simulink model "wind_disturbance"  (R2016b)
settings: Solver=VariableStepAuto  StartTime=0.0  StopTime=10.0  RelTol=1e-3
values from neighbouring files (symbols this model uses):
  K = gain(x)    [radar_sweep.m]    (also in sweep.m; sweep_1.m; sweep_2.m; wind_sweep.m)
settings Model: Creator=ammar_laptop  LastModifiedBy=ammar_laptop

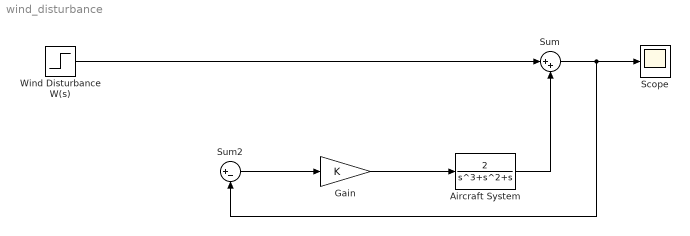
== system wind_disturbance ==
  Aircraft System : TransferFcn  Numerator=[2]  Denominator=[1 1 1 0]
  Gain : Gain  Gain=K
  Scope : Scope
  Sum : Sum  Inputs=|++
  Sum2 : Sum  Inputs=|+-
  Wind Disturbance W(s) : Step  SampleTime=0
  wires:
  Wind Disturbance W(s)/1 -> Sum/1
  Gain/1 -> Aircraft System/1
  Aircraft System/1 -> Sum/2
  Sum2/1 -> Gain/1
  Sum/1 -> Sum2/2, Scope/1
